simulink model "quadruped_robot"  (R2021a)
settings: Solver=ode15s  StartTime=0.0  StopTime=50  EnableMultiTasking=on
undefined symbols (not defined in the file): C, com_initial_height, H, joint_initial_q, L, L1, L2, L3, P0s, pc01, pc02, pc03, pc04, q0_leg1, q0_leg2, q0_leg3, q0_leg4, X, Y, Z
libraries: sm_lib x208, nesl_utility x124, roblocks x24, simulink_extras x5, pid_lib x2
(part 10 of 10)

== matlab function quadruped_robot/old_recalculate_legs_position ==
  data: u_rpy input; new_leg_pos output; legs_pos input; pb01 parameter; pb02 parameter; pb03 parameter; pb04 parameter
function new_leg_pos  = recalculate_legs_position(u_rpy, legs_pos, pb01, pb02, pb03, pb04)        

u_roll = u_rpy(1);
u_pitch = u_rpy(2);
u_yaw = u_rpy(3);

leg_1_pos = [legs_pos(1); legs_pos(2); legs_pos(3)];
leg_2_pos = [legs_pos(4); legs_pos(5); legs_pos(6)];
leg_3_pos = [legs_pos(7); legs_pos(8); legs_pos(9)];
leg_4_pos = [legs_pos(10); legs_pos(11); legs_pos(12)];


Rworld_base = rotx(rad2deg(u_roll))*roty(rad2deg(u_pitch))*rotz(rad2deg(u_yaw));

pos_base_1 = pb01(1:3,4);
pos_base_2 = pb02(1:3,4);
pos_base_3 = pb03(1:3,4);
pos_base_4 = pb04(1:3,4);

new_leg_1_pos = Rworld_base \ (leg_1_pos - pos_base_1) + pos_base_1;
new_leg_2_pos = Rworld_base \ (leg_2_pos - pos_base_2) + pos_base_2;
new_leg_3_pos = Rworld_base \ (leg_3_pos - pos_base_3) + pos_base_3;
new_leg_4_pos = Rworld_base \ (leg_4_pos - pos_base_4) + pos_base_4;

new_leg_pos = [new_leg_1_pos; new_leg_2_pos; new_leg_3_pos; new_leg_4_pos];

% fprintf('Roll: %.2f, Pitch: %.2f, Yaw: %.2f\n', rad2deg(u_roll), rad2deg(u_pitch), rad2deg(u_yaw));
% fprintf('Rworld_base:\n');
% fprintf('[%.3f %.3f %.3f]\n', Rworld_base(1,1), Rworld_base(1,2), Rworld_base(1,3));
% fprintf('[%.3f %.3f %.3f]\n', Rworld_base(2,1), Rworld_base(2,2), Rworld_base(2,3));
% fprintf('[%.3f %.3f %.3f]\n', Rworld_base(3,1), Rworld_base(3,2), Rworld_base(3,3));
% 
% fprintf('leg_1_pos: [%.3f %.3f %.3f]\n', leg_1_pos(1), leg_1_pos(2), leg_1_pos(3));
% fprintf('pos_base_1: [%.3f %.3f %.3f]\n', pos_base_1(1), pos_base_1(2), pos_base_1(3));
% fprintf('New Leg 1 Pos: [%.3f %.3f %.3f]\n', new_leg_1_pos(1), new_leg_1_pos(2), new_leg_1_pos(3));

== matlab function quadruped_robot/recalculate_legs_position ==
  data: u_rpy input; new_leg_pos output; legs_pos input; posCOM_W input
function new_leg_pos = recalculate_legs_position(u_rpy, legs_pos, posCOM_W)
% u_rpy = [roll; pitch; yaw]  (rad)
% legs_pos = [x1; y1; z1; x2; …] em frame mundo W
% posCOM_W = [x; y; z]  (centro do tronco em W)

roll  = u_rpy(1);
pitch = u_rpy(2);
yaw = u_rpy(3);

% Matriz que DESinclina
% R_nivel = rotx(rad2deg( roll )) * roty(rad2deg( pitch )); % apenas roll & pitch
R_nivel = rotx(rad2deg( roll )) * roty(rad2deg( pitch )) * rotz(rad2deg( yaw )); % roll, pitch e yaw

new_leg_pos = zeros(12,1);
for k = 1:4
    idx  = 3*(k-1)+(1:3);        % índices 1:3 4:6 …
    v_W  = legs_pos(idx) - posCOM_W;   % COM → pé
    v_B  = R_nivel \ v_W;               % remove só roll/pitch
    new_leg_pos(idx) = posCOM_W + v_B;  % alvo no mundo
end
end

== matlab function quadruped_robot/inverse_kinematics_analytical ==
  data: legs_pos input; legs_theta output; L_vec parameter; P0 parameter
function legs_theta = inverse_kinematics_analytical(legs_pos, L_vec, P0)
%#codegen
% legs_pos : 12x1  [x1;y1;z1; … x4;y4;z4]  (frame mundo)
% L_vec    : 1x3   [L1 L2 L3]
% P0       : 4x3   [p01; p02; p03; p04]  (origens no frame corpo)

L1 = L_vec(1);  L2 = L_vec(2);  L3 = L_vec(3);

legs_theta = zeros(12,1);   % saída pre-alocada

for i = 1:4
    %----------------------------------------------------------------------
    % 1. Extrai posição do pé i e origem da perna i
    %----------------------------------------------------------------------
    idx  = 3*(i-1)+(1:3);          % 1:3, 4:6, …
    pos  = legs_pos(idx);          % [xi; yi; zi]
    p0   = P0(i,:).';              % coluna [x0; y0; z0]
    
    %----------------------------------------------------------------------
    % 2. Plano Y-Z  (visão frontal)  → obtém θ1
    %----------------------------------------------------------------------
    n = abs(pos(2) - p0(2));       % |y - y0|
    m = abs(pos(3) - p0(3));       % |z - z0|
    p = sqrt(n*n + m*m);           % hipotenusa no plano
    beta = atan2(n,m);             % β
    tau  = asin( min(max(L1/p,-1),1) );   % τ  (clamp p≥L1)
    theta1 = beta - tau;           % θ1
    
    %----------------------------------------------------------------------
    % 3. Plano X-Z (visão lateral) → obtém θ2, θ3
    %----------------------------------------------------------------------
    R = sqrt(max(p*p - L1*L1, 0)); % distância do 2º joint ao pé
    b = pos(1) - p0(1);            % projeção em X
    c = R;                         % projeção em Z
    a = sqrt(b*b + c*c);           % dist. do joelho ao pé
    
    phi  = asin( min(max(b/a,-1),1) );
    alpha = acos( min(max((a*a + L2*L2 - L3*L3)/(2*a*L2),-1),1) );
    theta2 =  alpha - phi;
    
    theta3 = -pi + acos( min(max((L2*L2 + L3*L3 - a*a)/(2*L2*L3),-1),1) );
    
    %----------------------------------------------------------------------
    % 4. Inverte sinal para pernas 3 e 4 (caso cinemática espelhada)
    %----------------------------------------------------------------------
    if i == 3 || i == 4
        theta1 = -theta1;
        theta2 = -theta2;
        theta3 = -theta3;
    end
    
    legs_theta(idx) = [theta1; theta2; theta3];
end
end

== matlab function quadruped_robot/inverse_kinematics_analytical1 ==
  data: legs_pos input; legs_theta output; L_vec parameter; P0 parameter
function legs_theta = inverse_kinematics_analytical(legs_pos, L_vec, P0)
%#codegen
% legs_pos : 12x1  [x1;y1;z1; … x4;y4;z4]  (frame mundo)
% L_vec    : 1x3   [L1 L2 L3]
% P0       : 4x3   [p01; p02; p03; p04]  (origens no frame corpo)

L1 = L_vec(1);  L2 = L_vec(2);  L3 = L_vec(3);

legs_theta = zeros(12,1);   % saída pre-alocada

for i = 1:4
    %----------------------------------------------------------------------
    % 1. Extrai posição do pé i e origem da perna i
    %----------------------------------------------------------------------
    idx  = 3*(i-1)+(1:3);          % 1:3, 4:6, …
    pos  = legs_pos(idx);          % [xi; yi; zi]
    p0   = P0(i,:).';              % coluna [x0; y0; z0]
    
    %----------------------------------------------------------------------
    % 2. Plano Y-Z  (visão frontal)  → obtém θ1
    %----------------------------------------------------------------------
    n = abs(pos(2) - p0(2));       % |y - y0|
    m = abs(pos(3) - p0(3));       % |z - z0|
    p = sqrt(n*n + m*m);           % hipotenusa no plano
    beta = atan2(n,m);             % β
    tau  = asin( min(max(L1/p,-1),1) );   % τ  (clamp p≥L1)
    theta1 = beta - tau;           % θ1
    
    %----------------------------------------------------------------------
    % 3. Plano X-Z (visão lateral) → obtém θ2, θ3
    %----------------------------------------------------------------------
    R = sqrt(max(p*p - L1*L1, 0)); % distância do 2º joint ao pé
    b = pos(1) - p0(1);            % projeção em X
    c = R;                         % projeção em Z
    a = sqrt(b*b + c*c);           % dist. do joelho ao pé
    
    phi  = asin( min(max(b/a,-1),1) );
    alpha = acos( min(max((a*a + L2*L2 - L3*L3)/(2*a*L2),-1),1) );
    theta2 =  alpha - phi;
    
    theta3 = -pi + acos( min(max((L2*L2 + L3*L3 - a*a)/(2*L2*L3),-1),1) );
    
    %----------------------------------------------------------------------
    % 4. Inverte sinal para pernas 3 e 4 (caso cinemática espelhada)
    %----------------------------------------------------------------------
    if i == 3 || i == 4
        theta1 = -theta1;
        theta2 = -theta2;
        theta3 = -theta3;
    end
    
    legs_theta(idx) = [theta1; theta2; theta3];
end
end

== matlab function quadruped_robot/Quadruped Robot System3/IMU/rot2rpy ==
  data: R input; rpy output
function rpy  = rot2rpy(R)
ypr = rotm2eul(R, 'ZYX');
rpy = flip(ypr); % in radians
end
